simulink model "api_call_control_signals"  (R2024a)
settings: Solver=FixedStepDiscrete  StartTime=0.0  StopTime=200.0  FixedStep=1  RelTol=1e-3
libraries: simulink x1
settings Model: PacingRate=0.500000  Creator=vdikan  LastModifiedBy=vdikan

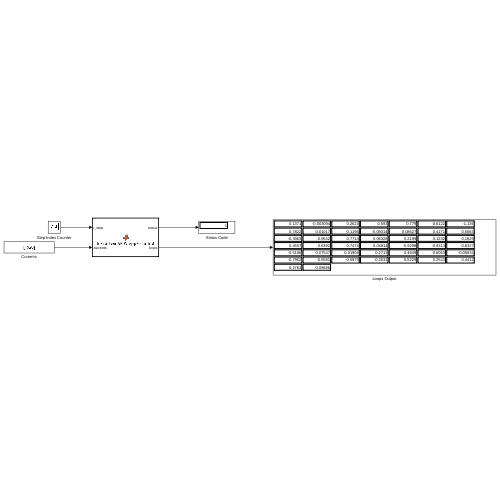
[thumbnail: Simulink's stored preview of the top-level diagram]
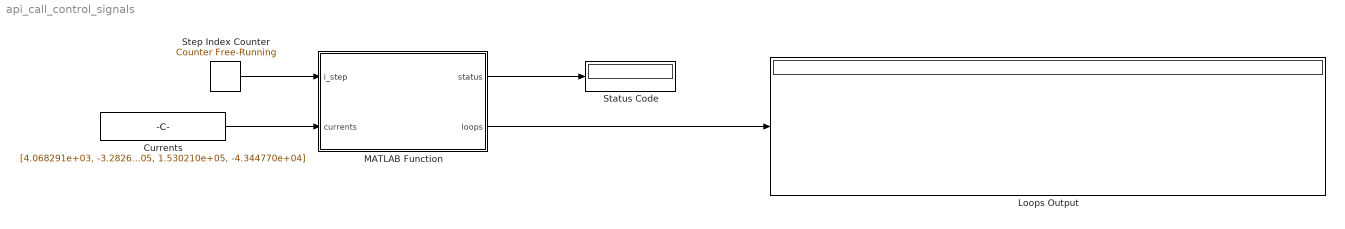
== system api_call_control_signals ==
  Currents : Constant  Value=[4.068291e+03, -3.282641e+03, -6.635891e+04, -1.695230e+05, -3.443223e+04, 1.140770e+05, 1.218360e+05, -1.560090e+05, -2.193246e+05, 1.248960e+05, -4.316320e+04, -6.181721e+04, -1.726810e+05, -4.876090e+04, 9.357561e+04, 5.540891e+04, -1.162780e+05, -1.989435e+05, 1.530210e+05, -4.344770e+04]
  Loops Output : Display
  MATLAB Function : MATLAB Function  TreatAsAtomicUnit=on
  Status Code : Display
  Step Index Counter : simulink/Sources/Counter Free-Running  NumBits=16  tsamp=-1
  wires:
  Step Index Counter/1 -> MATLAB Function/1(i_step)
  MATLAB Function/1(status) -> Status Code/1
  MATLAB Function/2(loops) -> Loops Output/1
  Currents/1 -> MATLAB Function/2(currents)

== matlab function api_call_control_signals/MATLAB Function ==
  data: status output; i_step input; loops output; currents input
function [status, loops] = fusionTwinAPIWrapperControl(i_step, currents)
    status = int8(0); loops = zeros(44,1);
    coder.extrinsic('fusiontwinapiwrappercontrol');
    [status, loops] = fusiontwinapiwrappercontrol(i_step, currents);
end
